simulink model "Braking_ABS"  (R2023b)
settings: Solver=VariableStepAuto  StartTime=0.0  StopTime=3  RelTol=1e-3
values from neighbouring files (symbols this model uses):
  A = 2    [Braking_Param.m]
  c1 = 0.86    [Braking_Param.m]
  c2 = 33.82    [Braking_Param.m]
  c3 = 0.36    [Braking_Param.m]
  cw = 0.3    [Braking_Param.m]
  g = 9.81    [Braking_Param.m]
  Jw = 0.8    [Braking_Param.m]
  Kc = 20000    [Braking_Param.m]
  m = 1500    [Braking_Param.m]
  p = 1.2    [Braking_Param.m]
  rw = 0.3    [Braking_Param.m]
  v0 = 100/3.6    (= 27.7777777778)    [Braking_Param.m]
settings Model: Creator=34266  LastModifiedBy=BeanieBabyJ
settings SolverCC: ZeroCrossAlgorithm=Adaptive
settings DebuggingCC: IgnoredZcDiagnostic=none

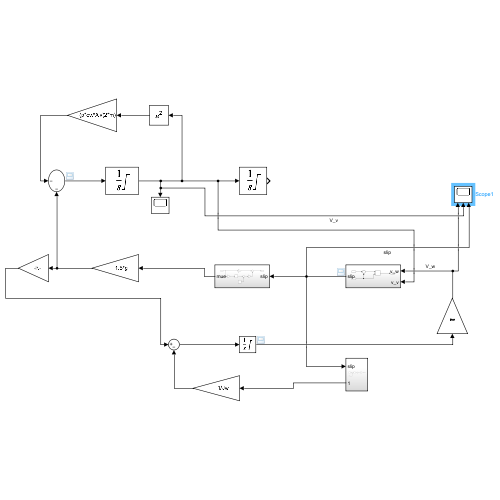
[thumbnail: Simulink's stored preview of the top-level diagram]
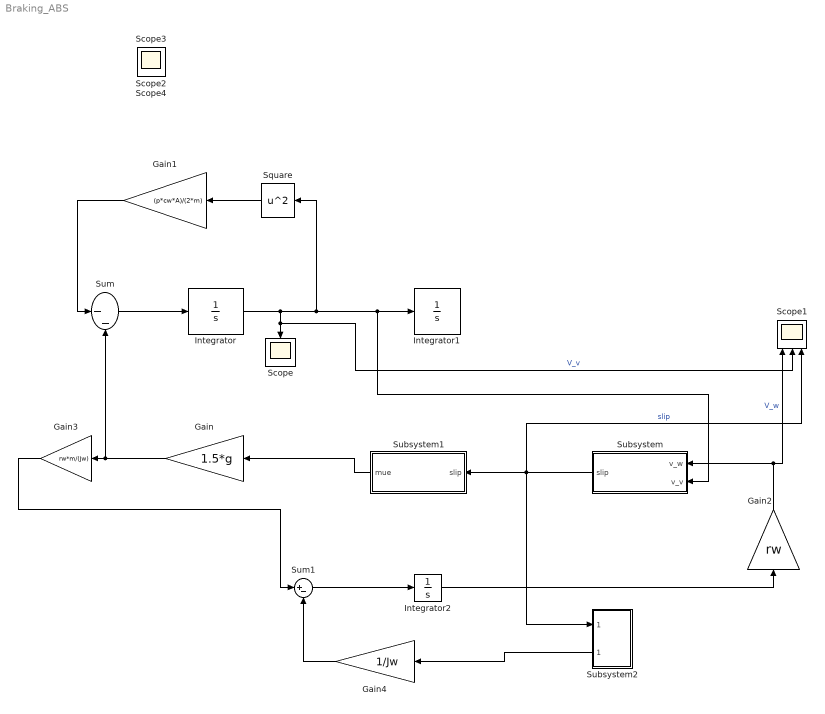
== system Braking_ABS ==
  Gain : Gain  Gain=1.5*g
  Gain1 : Gain  Gain=(p*cw*A)/(2*m)
  Gain2 : Gain  Gain=rw
  Gain3 : Gain  Gain=rw*m/(Jw)
  Gain4 : Gain  Gain=1/Jw
  Integrator : Integrator  InitialCondition=v0  LimitOutput=on  LowerSaturationLimit=0  ZeroCross=off
  Integrator1 : Integrator  LimitOutput=on  LowerSaturationLimit=0  ZeroCross=off
  Integrator2 : Integrator  InitialCondition=v0/rw  LimitOutput=on  LowerSaturationLimit=0  ZeroCross=off
  Scope{,2..4} (4 alike) : Scope
  Scope1 : Scope  NumInputPorts=3
  Square : Math  Operator=square
  Subsystem : Subsystem
  Subsystem1 : Subsystem
  Subsystem2 : Subsystem
      settings: PortSchema="{\"entries\":[{\"content\":{\"sides\":[{\"content\":{\"connectorIds\":[\"In1\",\"Out1\"]},\"type\":\"ConnectorPlacement.EquallySpacedRectSide\",\"uuid\":\"c8d10a41-c703-4ae3-9a55-6ad75991b8ec\"},{\"content\":{\"side\":\"RIGHT\"},\"type\":\"ConnectorPlacement.EquallySpacedRectSide\",\"uuid\":\"4f23f97a-b193-456e-912a-a2274241b3c8\"},{\"content\":{\"side\":\"TOP\"},\"type\":\"ConnectorPlacement.EquallySpacedRectSide\",\"uuid\":\"2ae19fe0-d5d7-40d7-abaf-d34ab4ff7945\"}]},\"type\":\"ConnectorPlacement.EquallySpacedConnector\",\"uuid\":\"251a3f80-cd5b-4f23-9272-cc2d9d8990b0\"}],\"packageUris\":[\"http://schema.mathworks.com/mf0/Connector/R2020b\"],\"version\":\"1.0\"}"
  Sum : Sum  Inputs=|--
  Sum1 : Sum  Inputs=|+-
  wires:
  Subsystem/1(slip) -> Subsystem2/1(slip), Scope1/3, Subsystem1/1(slip)  "slip"
  Integrator/1 -> Scope1/2, Scope/1, Square/1, Subsystem/2(v_v), Integrator1/1  "V_v"
  Sum/1 -> Integrator/1
  Gain/1 -> Gain3/1, Sum/2
  Subsystem1/1(mue) -> Gain/1
  Gain1/1 -> Sum/1
  Square/1 -> Gain1/1
  Sum1/1 -> Integrator2/1
  Subsystem2/1(Out1) -> Gain4/1
  Gain3/1 -> Sum1/1
  Integrator2/1 -> Gain2/1
  Gain2/1 -> Subsystem/1(v_w), Scope1/1  "V_w"
  Gain4/1 -> Sum1/2

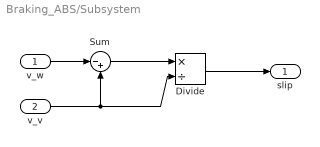
== system Braking_ABS/Subsystem ==
  v_w : Inport
  v_v : Inport  Port=2
  Divide : Product  Inputs=*/
  Sum : Sum  Inputs=|-+
  slip : Outport
  wires:
  Sum/1 -> Divide/1
  v_v/1 -> Sum/2, Divide/2
  v_w/1 -> Sum/1
  Divide/1 -> slip/1

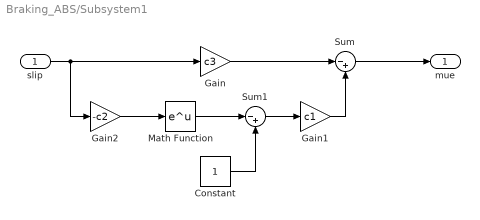
== system Braking_ABS/Subsystem1 ==
  slip : Inport
  Constant : Constant
  Gain : Gain  Gain=c3
  Gain1 : Gain  Gain=c1
  Gain2 : Gain  Gain=-c2
  Math Function : Math
  Sum : Sum  Inputs=|-+
  Sum1 : Sum  Inputs=|-+
  mue : Outport
  wires:
  Sum1/1 -> Gain1/1
  slip/1 -> Gain/1, Gain2/1
  Gain2/1 -> Math Function/1
  Math Function/1 -> Sum1/1
  Constant/1 -> Sum1/2
  Gain1/1 -> Sum/2
  Gain/1 -> Sum/1
  Sum/1 -> mue/1

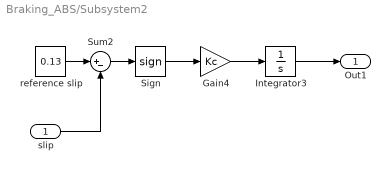
== system Braking_ABS/Subsystem2 ==
  slip : Inport
  Gain4 : Gain  Gain=Kc
  Integrator3 : Integrator  LimitOutput=on  LowerSaturationLimit=0  ZeroCross=off
  Sign : Signum
  Sum2 : Sum  Inputs=|+-
  reference slip : Constant  Value=0.13
  Out1 : Outport
  wires:
  Gain4/1 -> Integrator3/1
  slip/1 -> Sum2/2
  Sum2/1 -> Sign/1
  Sign/1 -> Gain4/1
  reference slip/1 -> Sum2/1
  Integrator3/1 -> Out1/1
